simulink model "turkp"  (R2023a)
settings: Solver=ode45  StartTime=0.0  StopTime=1  RelTol=1e-6  EnableMultiTasking=on
settings Model: Creator=Пользователь  LastModifiedBy=k.balkunov
settings SolverCC: AlgebraicLoopSolver=TrustRegion
settings DataIOCC: LimitDataPoints=on  SaveFormat=Array  ReturnWorkspaceOutputs=off
settings OptimizationCC: ExpressionDepthLimit=2147483647  LifeSpan=inf
settings DebuggingCC: UnderspecifiedInitializationDetection=Classic  MergeDetectMultiDrivingBlocksExec=none  SolverPrmCheckMsg=warning  UnconnectedInputMsg=warning  UnconnectedOutputMsg=warning  UnconnectedLineMsg=warning  StateNameClashWarn=warning  SFUnexpectedBacktrackingDiag=warning  SFNoUnconditionalDefaultTransitionDiag=warning  SFExecutionAtInitializationDiag=none  ArithmeticOperatorsInVariantConditions=warning
settings HardwareCC: ProdBitPerPointer=32  ProdBitPerSizeT=32  ProdBitPerPtrDiffT=32  ProdLargestAtomicFloat=None  ProdIntDivRoundTo=Undefined  ProdEndianess=Unspecified  ProdWordSize=32  ProdHWDeviceType=32-bit Generic
settings ModelReferenceCC: PropagateSignalLabelsOutOfModel=off
settings SFSimCC: SimUseLocalCustomCode=off  CustomCodeUndefinedFunction=UseInterfaceOnly
settings RTWCC: RTWUseLocalCustomCode=off
settings CodeAppCC: StateflowObjectComments=on
settings GRTTargetCC: TargetLangStandard=C89/C90 (ANSI)
settings ConfigComp: CovMetricSettings=dw  CovSaveCumulativeToWorkspaceVar=on  CovSaveSingleToWorkspaceVar=on  CovExternalEMLEnable=off

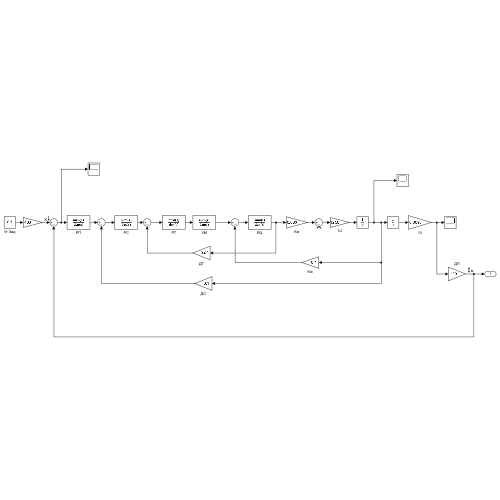
[thumbnail: Simulink's stored preview of the top-level diagram]
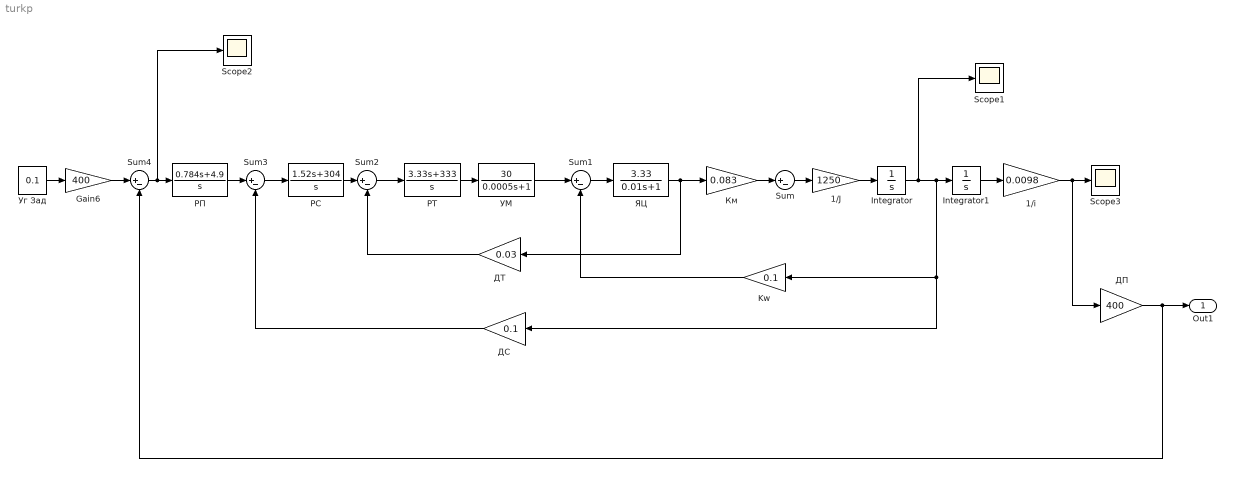
== system turkp ==
  1/J : Gain  Gain=1250
  1/i : Gain  Gain=0.0098
  Gain6 : Gain  Gain=400
  Integrator : Integrator
  Integrator1 : Integrator
  Kw : Gain  Gain=0.1
  Scope1 : Scope
  Scope2 : Scope
  Scope3 : Scope
  Sum{,1..4} (5 alike) : Sum  Inputs=|+-
  ДП : Gain  Gain=400
  ДС : Gain  Gain=0.1
  ДТ : Gain  Gain=0.03
  Км : Gain  Gain=0.083
  РП : TransferFcn  Numerator=[0.784 4.9]  Denominator=[1 0]
  РС : TransferFcn  Numerator=[1.52 304]  Denominator=[1 0]
  РТ : TransferFcn  Numerator=[3.33 333]  Denominator=[1 0]
  УМ : TransferFcn  Numerator=[30]  Denominator=[0.0005 1]
  Уг Зад : Constant  Value=0.1
  ЯЦ : TransferFcn  Numerator=[3.33]  Denominator=[0.01 1]
  Out1 : Outport
  wires:
  Sum1/1 -> ЯЦ/1
  Км/1 -> Sum/1
  Sum/1 -> 1/J/1
  1/J/1 -> Integrator/1
  Integrator/1 -> Scope1/1, Integrator1/1, ДС/1, Kw/1
  УМ/1 -> Sum1/1
  Sum2/1 -> РТ/1
  ЯЦ/1 -> ДТ/1, Км/1
  Kw/1 -> Sum1/2
  РТ/1 -> УМ/1
  Sum3/1 -> РС/1
  РС/1 -> Sum2/1
  ДТ/1 -> Sum2/2
  ДС/1 -> Sum3/2
  РП/1 -> Sum3/1
  Sum4/1 -> Scope2/1, РП/1
  Integrator1/1 -> 1/i/1
  1/i/1 -> Scope3/1, ДП/1
  Gain6/1 -> Sum4/1
  Уг Зад/1 -> Gain6/1
  ДП/1 -> Sum4/2, Out1/1
